simulink model "CIUDAT"  (R2014b)
settings: Solver=ode45  StartTime=0.0  StopTime=150  RelTol=1e-3
values from neighbouring files (symbols this model uses):
  Th_coefOmega_e = (omega_e-4070.3)/0.2685    [liniarizare_crazyflie.m]
undefined symbols (not defined in the file or in its folder): A, B, C, D
libraries: simulink x5
settings Model: Creator=uidd7441  LastModifiedBy=uidd7441

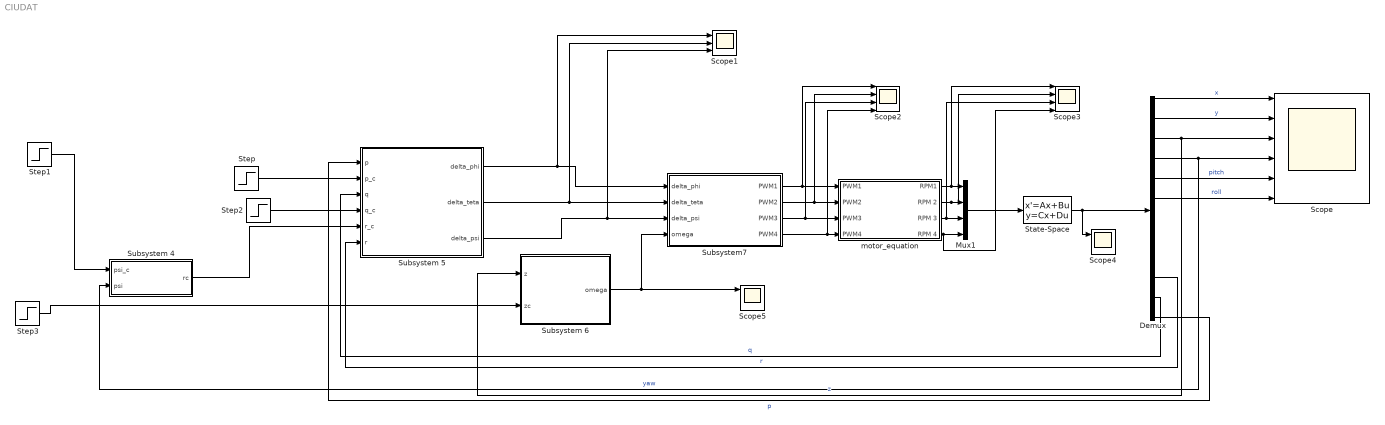
== system CIUDAT ==
  Demux : Demux  Outputs=12
  Mux1 : Mux
  Scope : Scope  NumInputPorts=6
      settings: YMin=-5~-5~-5~-5~-5~-5  YMax=5~5~5~5~5~5
  Scope1 : Scope  NumInputPorts=3
      settings: YMin=-5~-5~-5  YMax=5~5~5  SaveName=ScopeData4
  Scope2 : Scope  NumInputPorts=4
      settings: YMin=-5~-5~-5~-5  YMax=5~5~5~5  SaveName=ScopeData5  SampleInput=on
  Scope3 : Scope  NumInputPorts=4
      settings: YMin=-5~-5~-5~-5  YMax=5~5~5~5  SaveName=ScopeData6  SampleInput=on
  Scope4 : Scope  NumInputPorts=3
      settings: YMin=-5~-5~-5  YMax=5~5~5  SaveName=ScopeData7
  Scope5 : Scope  NumInputPorts=3
      settings: YMin=-5~-5~-5  YMax=5~5~5  SaveName=ScopeData8
  State-Space : StateSpace  A=A  B=B  C=C  D=D  X0=[0 0 0 0 0 0 0 0 0 0 0 0]
  Step : Step  Time=0  After=0.001  SampleTime=0
  Step1 : Step  Time=0  SampleTime=0
  Step2 : Step  Time=0  After=0  SampleTime=0
  Step3 : Step  Time=0  After=5  SampleTime=0
  Subsystem 4 : Subsystem
  Subsystem 5 : Subsystem
  Subsystem 6 : Subsystem
  Subsystem7 : Subsystem
  motor_equation : Subsystem
  wires:
  Subsystem 4/1(rc) -> Subsystem 5/5(r_c)
  Subsystem 6/1(omega) -> Subsystem7/4(omega), Scope5/1
  Subsystem7/1(PWM1) -> Scope2/1, motor_equation/1(PWM1)
  Subsystem7/2(PWM2) -> Scope2/2, motor_equation/2(PWM2)
  Subsystem7/3(PWM3) -> Scope2/3, motor_equation/3(PWM3)
  Subsystem7/4(PWM4) -> Scope2/4, motor_equation/4(PWM4)
  State-Space/1 -> Scope4/1, Demux/1
  motor_equation/1("RPM1 ") -> Scope3/1, Mux1/1
  motor_equation/2(RPM 2) -> Scope3/2, Mux1/2
  motor_equation/3(RPM 3) -> Mux1/3, Scope3/3
  motor_equation/4(RPM 4) -> Scope3/4, Mux1/4
  Mux1/1 -> State-Space/1
  Demux/11 -> Subsystem 5/3(q)  "q"
  Demux/10 -> Subsystem 5/6(r)  "r"
  Subsystem 5/1(delta_phi) -> Scope1/1, Subsystem7/1(delta_phi)
  Subsystem 5/2(delta_teta) -> Scope1/2, Subsystem7/2(delta_teta)
  Step/1 -> Subsystem 5/2(p_c)
  Demux/1 -> Scope/1  "x"
  Demux/2 -> Scope/2  "y"
  Demux/3 -> Subsystem 6/1(z), Scope/3  "z"
  Demux/4 -> Subsystem 4/2(psi), Scope/4  "yaw"
  Demux/5 -> Scope/5  "pitch"
  Demux/6 -> Scope/6  "roll"
  Step1/1 -> Subsystem 4/1(psi_c)
  Step2/1 -> Subsystem 5/4(q_c)
  Step3/1 -> Subsystem 6/2(zc)
  Subsystem 5/3(delta_psi) -> Scope1/3, Subsystem7/3(delta_psi)
  Demux/12 -> Subsystem 5/1(p)  "p"

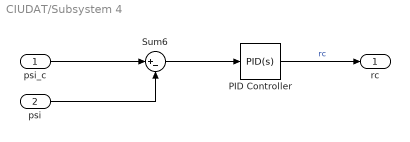
== system CIUDAT/Subsystem 4 ==
  psi_c : Inport
  psi : Inport  Port=2
  PID Controller : simulink/Continuous/PID Controller  Controller=PID  TimeDomain=Continuous-time  SampleTime=-1  IntegratorMethod=Forward Euler  FilterMethod=Forward Euler  Form=Parallel  P=3  I=0  D=0  N=0  InitialConditionSource=internal  InitialConditionForIntegrator=0  InitialConditionForFilter=0  ExternalReset=none  LimitOutput=off  UpperSaturationLimit=200  LowerSaturationLimit=-200  LinearizeAsGain=on  AntiWindupMode=none  Kb=1  TrackingMode=off  Kt=1  PParamMin=[]  PParamMax=[]  IParamMin=[]  IParamMax=[]  DParamMin=[]  DParamMax=[]  NParamMin=[]  NParamMax=[]  KbParamMin=[]  KbParamMax=[]  KtParamMin=[]  KtParamMax=[]  POutMin=[]  POutMax=[]  IOutMin=[]  IOutMax=[]  DOutMin=[]  DOutMax=[]  NOutMin=[]  NOutMax=[]  KbOutMin=[]  KbOutMax=[]  KtOutMin=[]  KtOutMax=[]  IntegratorOutMin=[]  IntegratorOutMax=[]  FilterOutMin=[]  FilterOutMax=[]  SumOutMin=[]  SumOutMax=[]  SumI1OutMin=[]  SumI1OutMax=[]  SumI2OutMin=[]  SumI2OutMax=[]  SumI3OutMin=[]  SumI3OutMax=[]  SumDOutMin=[]  SumDOutMax=[]  SaturationOutMin=[]  SaturationOutMax=[]  IntegratorContinuousStateAttributes=''  IntegratorStateMustResolveToSignalObject=off  IntegratorRTWStateStorageClass=Auto  FilterContinuousStateAttributes=''  FilterStateMustResolveToSignalObject=off  FilterRTWStateStorageClass=Auto  DifferentiatorICPrevScaledInput=0  DifferentiatorOutMin=[]  DifferentiatorOutMax=[]  UseFilter=on
  Sum6 : Sum  Inputs=|+-
  rc : Outport
  wires:
  Sum6/1 -> PID Controller/1
  PID Controller/1 -> rc/1  "rc"
  psi_c/1 -> Sum6/1
  psi/1 -> Sum6/2

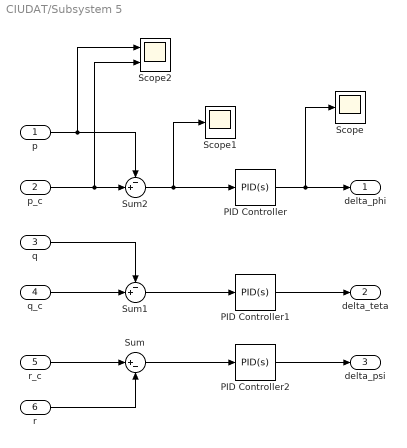
== system CIUDAT/Subsystem 5 ==
  p : Inport
  p_c : Inport  Port=2
  q : Inport  Port=3
  q_c : Inport  Port=4
  r_c : Inport  Port=5
  r : Inport  Port=6
  PID Controller : simulink/Continuous/PID Controller  Controller=PID  TimeDomain=Continuous-time  SampleTime=-1  IntegratorMethod=Forward Euler  FilterMethod=Forward Euler  Form=Parallel  P=70  I=0  D=0  N=100  InitialConditionSource=internal  InitialConditionForIntegrator=0  InitialConditionForFilter=0  ExternalReset=none  LimitOutput=off  UpperSaturationLimit=inf  LowerSaturationLimit=-inf  LinearizeAsGain=on  AntiWindupMode=none  Kb=1  TrackingMode=off  Kt=1  PParamMin=[]  PParamMax=[]  IParamMin=[]  IParamMax=[]  DParamMin=[]  DParamMax=[]  NParamMin=[]  NParamMax=[]  KbParamMin=[]  KbParamMax=[]  KtParamMin=[]  KtParamMax=[]  POutMin=[]  POutMax=[]  IOutMin=[]  IOutMax=[]  DOutMin=[]  DOutMax=[]  NOutMin=[]  NOutMax=[]  KbOutMin=[]  KbOutMax=[]  KtOutMin=[]  KtOutMax=[]  IntegratorOutMin=[]  IntegratorOutMax=[]  FilterOutMin=[]  FilterOutMax=[]  SumOutMin=[]  SumOutMax=[]  SumI1OutMin=[]  SumI1OutMax=[]  SumI2OutMin=[]  SumI2OutMax=[]  SumI3OutMin=[]  SumI3OutMax=[]  SumDOutMin=[]  SumDOutMax=[]  SaturationOutMin=[]  SaturationOutMax=[]  IntegratorContinuousStateAttributes=''  IntegratorStateMustResolveToSignalObject=off  IntegratorRTWStateStorageClass=Auto  FilterContinuousStateAttributes=''  FilterStateMustResolveToSignalObject=off  FilterRTWStateStorageClass=Auto  DifferentiatorICPrevScaledInput=0  DifferentiatorOutMin=[]  DifferentiatorOutMax=[]  UseFilter=on
  PID Controller1 : simulink/Continuous/PID Controller  Controller=PID  TimeDomain=Continuous-time  SampleTime=-1  IntegratorMethod=Forward Euler  FilterMethod=Forward Euler  Form=Parallel  P=70  I=0  D=0  N=100  InitialConditionSource=internal  InitialConditionForIntegrator=0  InitialConditionForFilter=0  ExternalReset=none  LimitOutput=off  UpperSaturationLimit=inf  LowerSaturationLimit=-inf  LinearizeAsGain=on  AntiWindupMode=none  Kb=1  TrackingMode=off  Kt=1  PParamMin=[]  PParamMax=[]  IParamMin=[]  IParamMax=[]  DParamMin=[]  DParamMax=[]  NParamMin=[]  NParamMax=[]  KbParamMin=[]  KbParamMax=[]  KtParamMin=[]  KtParamMax=[]  POutMin=[]  POutMax=[]  IOutMin=[]  IOutMax=[]  DOutMin=[]  DOutMax=[]  NOutMin=[]  NOutMax=[]  KbOutMin=[]  KbOutMax=[]  KtOutMin=[]  KtOutMax=[]  IntegratorOutMin=[]  IntegratorOutMax=[]  FilterOutMin=[]  FilterOutMax=[]  SumOutMin=[]  SumOutMax=[]  SumI1OutMin=[]  SumI1OutMax=[]  SumI2OutMin=[]  SumI2OutMax=[]  SumI3OutMin=[]  SumI3OutMax=[]  SumDOutMin=[]  SumDOutMax=[]  SaturationOutMin=[]  SaturationOutMax=[]  IntegratorContinuousStateAttributes=''  IntegratorStateMustResolveToSignalObject=off  IntegratorRTWStateStorageClass=Auto  FilterContinuousStateAttributes=''  FilterStateMustResolveToSignalObject=off  FilterRTWStateStorageClass=Auto  DifferentiatorICPrevScaledInput=0  DifferentiatorOutMin=[]  DifferentiatorOutMax=[]  UseFilter=on
  PID Controller2 : simulink/Continuous/PID Controller  Controller=PID  TimeDomain=Continuous-time  SampleTime=-1  IntegratorMethod=Forward Euler  FilterMethod=Forward Euler  Form=Parallel  P=70  I=16.7  D=0  N=100  InitialConditionSource=internal  InitialConditionForIntegrator=0  InitialConditionForFilter=0  ExternalReset=none  LimitOutput=off  UpperSaturationLimit=inf  LowerSaturationLimit=-inf  LinearizeAsGain=on  AntiWindupMode=none  Kb=1  TrackingMode=off  Kt=1  PParamMin=[]  PParamMax=[]  IParamMin=[]  IParamMax=[]  DParamMin=[]  DParamMax=[]  NParamMin=[]  NParamMax=[]  KbParamMin=[]  KbParamMax=[]  KtParamMin=[]  KtParamMax=[]  POutMin=[]  POutMax=[]  IOutMin=[]  IOutMax=[]  DOutMin=[]  DOutMax=[]  NOutMin=[]  NOutMax=[]  KbOutMin=[]  KbOutMax=[]  KtOutMin=[]  KtOutMax=[]  IntegratorOutMin=[]  IntegratorOutMax=[]  FilterOutMin=[]  FilterOutMax=[]  SumOutMin=[]  SumOutMax=[]  SumI1OutMin=[]  SumI1OutMax=[]  SumI2OutMin=[]  SumI2OutMax=[]  SumI3OutMin=[]  SumI3OutMax=[]  SumDOutMin=[]  SumDOutMax=[]  SaturationOutMin=[]  SaturationOutMax=[]  IntegratorContinuousStateAttributes=''  IntegratorStateMustResolveToSignalObject=off  IntegratorRTWStateStorageClass=Auto  FilterContinuousStateAttributes=''  FilterStateMustResolveToSignalObject=off  FilterRTWStateStorageClass=Auto  DifferentiatorICPrevScaledInput=0  DifferentiatorOutMin=[]  DifferentiatorOutMax=[]  UseFilter=on
  Scope : Scope
  Scope1 : Scope
      settings: SaveName=ScopeData2
  Scope2 : Scope  NumInputPorts=2
      settings: YMin=-5~-5  YMax=5~5  SaveName=ScopeData3  SampleInput=on
  Sum : Sum  Inputs=|+-
  Sum1 : Sum  Inputs=-+|
  Sum2 : Sum  Inputs=-+|
  delta_phi : Outport
  delta_teta : Outport  Port=2
  delta_psi : Outport  Port=3
  wires:
  q/1 -> Sum1/1
  q_c/1 -> Sum1/2
  p_c/1 -> Scope2/2, Sum2/2
  p/1 -> Scope2/1, Sum2/1
  r_c/1 -> Sum/1
  r/1 -> Sum/2
  Sum2/1 -> Scope1/1, PID Controller/1
  Sum1/1 -> PID Controller1/1
  Sum/1 -> PID Controller2/1
  PID Controller/1 -> Scope/1, delta_phi/1
  PID Controller1/1 -> delta_teta/1
  PID Controller2/1 -> delta_psi/1

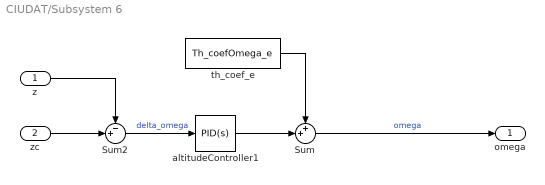
== system CIUDAT/Subsystem 6 ==
  z : Inport
  zc : Inport  Port=2
  Sum : Sum  Inputs=++|
  Sum2 : Sum  Inputs=-+|
  altitudeController1 : simulink/Continuous/PID Controller  Controller=PID  TimeDomain=Continuous-time  SampleTime=-1  IntegratorMethod=Forward Euler  FilterMethod=Forward Euler  Form=Parallel  P=11000  I=3500  D=9000  N=100  InitialConditionSource=internal  InitialConditionForIntegrator=0  InitialConditionForFilter=0  ExternalReset=none  LimitOutput=off  UpperSaturationLimit=20000  LowerSaturationLimit=-15000  LinearizeAsGain=on  AntiWindupMode=none  Kb=1  TrackingMode=off  Kt=1  PParamMin=[]  PParamMax=[]  IParamMin=[]  IParamMax=[]  DParamMin=[]  DParamMax=[]  NParamMin=[]  NParamMax=[]  KbParamMin=[]  KbParamMax=[]  KtParamMin=[]  KtParamMax=[]  POutMin=[]  POutMax=[]  IOutMin=[]  IOutMax=[]  DOutMin=[]  DOutMax=[]  NOutMin=[]  NOutMax=[]  KbOutMin=[]  KbOutMax=[]  KtOutMin=[]  KtOutMax=[]  IntegratorOutMin=[]  IntegratorOutMax=[]  FilterOutMin=[]  FilterOutMax=[]  SumOutMin=[]  SumOutMax=[]  SumI1OutMin=[]  SumI1OutMax=[]  SumI2OutMin=[]  SumI2OutMax=[]  SumI3OutMin=[]  SumI3OutMax=[]  SumDOutMin=[]  SumDOutMax=[]  SaturationOutMin=[]  SaturationOutMax=[]  IntegratorContinuousStateAttributes=''  IntegratorStateMustResolveToSignalObject=off  IntegratorRTWStateStorageClass=Auto  FilterContinuousStateAttributes=''  FilterStateMustResolveToSignalObject=off  FilterRTWStateStorageClass=Auto  DifferentiatorICPrevScaledInput=0  DifferentiatorOutMin=[]  DifferentiatorOutMax=[]  UseFilter=on
  "th_coef_e " : Constant  Value=Th_coefOmega_e
  omega : Outport
  wires:
  "th_coef_e "/1 -> Sum/1
  Sum/1 -> omega/1  "omega"
  zc/1 -> Sum2/2
  z/1 -> Sum2/1
  Sum2/1 -> altitudeController1/1  "delta_omega"
  altitudeController1/1 -> Sum/2

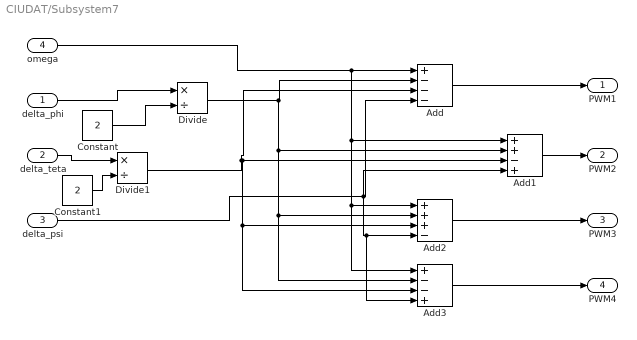
== system CIUDAT/Subsystem7 ==
  delta_phi : Inport
  delta_teta : Inport  Port=2
  delta_psi : Inport  Port=3
  omega : Inport  Port=4
  Add : Sum  Inputs=+---
  Add1 : Sum  Inputs=++-+
  Add2 : Sum  Inputs=+++-
  Add3 : Sum  Inputs=+--+
  Constant : Constant  Value=2
  Constant1 : Constant  Value=2
  Divide : Product  Inputs=*/
  Divide1 : Product  Inputs=*/
  PWM1 : Outport
  PWM2 : Outport  Port=2
  PWM3 : Outport  Port=3
  PWM4 : Outport  Port=4
  wires:
  delta_phi/1 -> Divide/1
  delta_teta/1 -> Divide1/1
  Add/1 -> PWM1/1
  Add1/1 -> PWM2/1
  Add2/1 -> PWM3/1
  Add3/1 -> PWM4/1
  omega/1 -> Add3/1, Add2/1, Add1/1, Add/1
  Divide/1 -> Add3/2, Add2/2, Add1/2, Add/2
  Divide1/1 -> Add/3, Add3/3, Add2/3, Add1/3
  delta_psi/1 -> Add3/4, Add2/4, Add1/4, Add/4
  Constant/1 -> Divide/2
  Constant1/1 -> Divide1/2

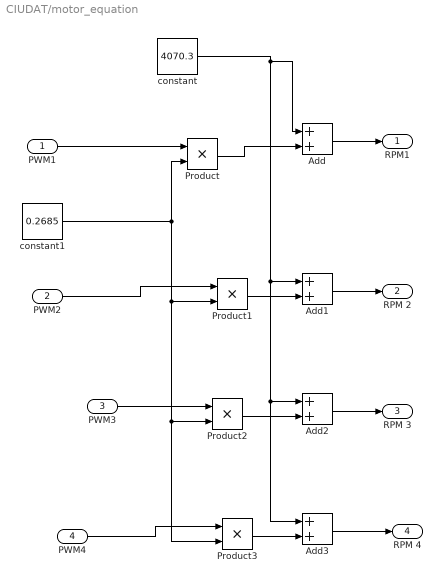
== system CIUDAT/motor_equation ==
  PWM1 : Inport
  PWM2 : Inport  Port=2
  PWM3 : Inport  Port=3
  PWM4 : Inport  Port=4
  Add{,1..3} (4 alike) : Sum
  Product{,1..3} (4 alike) : Product
  constant : Constant  Value=4070.3
  constant1 : Constant  Value=0.2685
  "RPM1 " : Outport
  RPM 2 : Outport  Port=2
  RPM 3 : Outport  Port=3
  RPM 4 : Outport  Port=4
  wires:
  constant/1 -> Add3/1, Add2/1, Add1/1, Add/1
  Product/1 -> Add/2
  PWM1/1 -> Product/1
  Add/1 -> "RPM1 "/1
  Product1/1 -> Add1/2
  PWM2/1 -> Product1/1
  Add1/1 -> RPM 2/1
  Product2/1 -> Add2/2
  PWM3/1 -> Product2/1
  Add2/1 -> RPM 3/1
  Product3/1 -> Add3/2
  PWM4/1 -> Product3/1
  Add3/1 -> RPM 4/1
  constant1/1 -> Product/2, Product3/2, Product2/2, Product1/2
